simulink model "stm32_system_identification"  (R2025a)
settings: Solver=VariableStepAuto  StartTime=0.0  StopTime=10.0  RelTol=1e-3
values from neighbouring files (symbols this model uses):
  motor_B = 0.000032047    (= 3.2047e-05)    [Lab1_motor_params_student.m]    (also in Params_Chirp.mat = 0.00100006396424; Params_Ramp.mat = 0.301544637419; Params_Sine.mat = 0.229979738857; Params_Stair.mat = 0.140998803706)
  motor_Eff = 0.952868616    [Lab1_motor_params_student.m]    (also in Params_Chirp.mat = 0.999510591885; Params_Ramp.mat = 0.511135750028; Params_Sine.mat = 1; Params_Stair.mat = 0.999629522012)
  motor_J = 0.000009875    (= 9.875e-06)    [Lab1_motor_params_student.m]    (also in Params_Chirp.mat = 0.00100180066555; Params_Ramp.mat = 0.35220653698; Params_Sine.mat = 0.261312099523; Params_Stair.mat = 0.298587602887)
  motor_Ke = 0.047996267    [Lab1_motor_params_student.m]    (also in Params_Chirp.mat = 0.574998179044; Params_Ramp.mat = 0.149481279538; Params_Sine.mat = 0.241485328515; Params_Stair.mat = 0.261815421338)
  motor_L = 0.002853248    [Lab1_motor_params_student.m]
  motor_R = 3.399924458    [Lab1_motor_params_student.m]
undefined symbols (not defined in the file or in its folder): Blocking, LF, Non
libraries: simulink x3, amg_usbconverter_n_connect_lib x3, dspstat3 x1
settings Model: Creator=User  LastModifiedBy=User

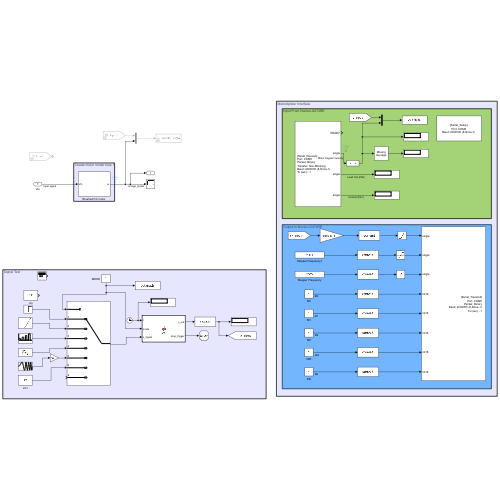
[thumbnail: Simulink's stored preview of the top-level diagram]
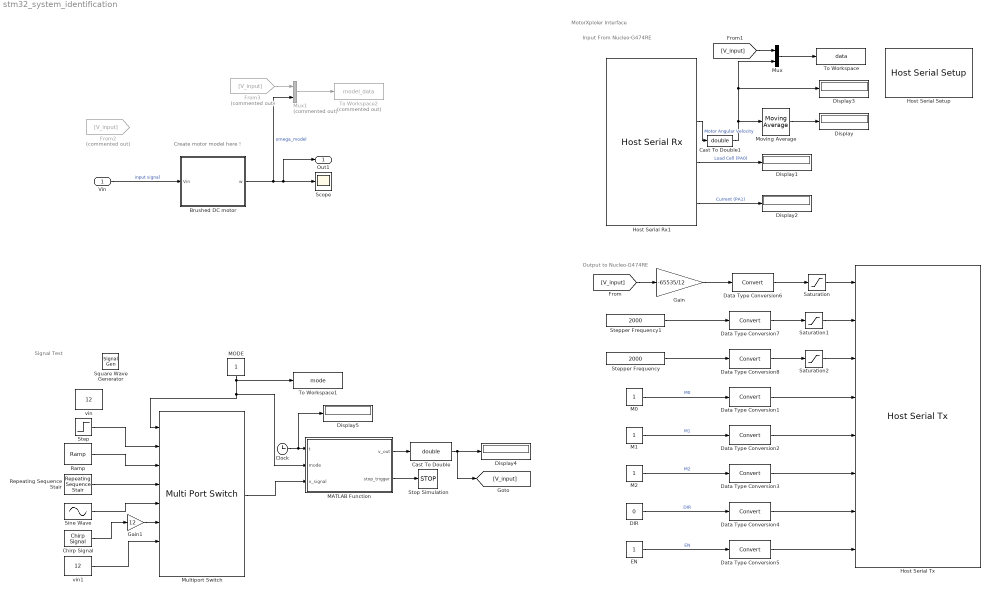
== system stm32_system_identification ==
  note: Signal Test
  note: Input From Nucleo-G474RE
  note: Output to Nucleo-G474RE
  note: MotorXploler Interface
  note: Create motor model here !
  Vin : Inport
  Brushed DC motor : Subsystem
  Cast To Double : DataTypeConversion  OutDataTypeStr=double  SaturateOnIntegerOverflow=off  RndMeth=Floor
  Cast To Double1 : DataTypeConversion  OutDataTypeStr=double  SaturateOnIntegerOverflow=off  RndMeth=Floor
  Chirp Signal : simulink/Sources/Chirp Signal  f1=0  T=20  f2=pi
  Clock : Clock
      settings: Decimation=5
  DIR : Constant  Value=0
  Data Type Conversion{1..8} (8 alike) : DataTypeConversion  SaturateOnIntegerOverflow=off  RndMeth=Floor
  Display{,1..5} (6 alike) : Display
  EN : Constant
  From2 : From  Commented=on  GotoTag=V_input
  From3 : From  Commented=on  GotoTag=V_input
  Gain : Gain  Gain=-65535/12
  Gain1 : Gain  Gain=12
  Host Serial Rx1 : amg_usbconverter_n_connect_lib/Host Serial Rx  conf=rx  port=<auto>  baudrate=2000000  databits=8  parity=None  stopbit=1  flowcontrol=None  transfer=Non-Blocking  timeout=5  packetmode=Binary  enableinitialvalues=off  initialvalues=[]  binheader='25'  binterminator='4E'  porttype_double=0  porttype_single=3  porttype_int8=0  porttype_uint8=0  porttype_int16=0  porttype_uint16=0  porttype_int32=0  porttype_uint32=0  asciiformat='%f,%f,%d,%d'  rx_asciiterminator="LF (0x0A - \"\\n\")"  tx_asciiterminator="CRLF (0x0D 0x0A - \"\\r\\n\")"  sampletime=-1  enablecustomportlabel=off  cinputportlabel=0  coutputportlabel=A  portpinstr=0  blockid=HostSerialRx1  inputporttype=[]  inputportwidth=[]  inputportlabel={}  outputporttype=[3 1 1 1]  outputportwidth=[1 1 1 1]  outputportlabel={'READY','single','single','single'}  compat=0  optionstring=[]  autoport='COM5'
  Host Serial Setup : amg_usbconverter_n_connect_lib/Host Serial Setup  conf=setup  port=<auto>  baudrate=2000000  databits=8  parity=None  stopbit=1  flowcontrol=None  transfer=Blocking  timeout=2  packetmode=Binary  initialvalues=[]  binheader='7E 7E'  binterminator='03 03'  porttype_double=0  porttype_single=1  porttype_int8=0  porttype_uint8=0  porttype_int16=0  porttype_uint16=0  porttype_int32=0  porttype_uint32=2  asciiformat='%d %u %x'  rx_asciiterminator="CRLF (0x0D 0x0A - \"\\r\\n\")"  tx_asciiterminator="CRLF (0x0D 0x0A - \"\\r\\n\")"  sampletime=-1  enablecustomportlabel=off  cinputportlabel=0  coutputportlabel=A  portpinstr=0  blockid=HostSerialSetup  inputporttype=[]  inputportwidth=[]  inputportlabel={}  outputporttype=[]  outputportwidth=[]  outputportlabel={}  compat=0  optionstring=[]  autoport='COM5'
  Host Serial Tx : amg_usbconverter_n_connect_lib/Host Serial Tx  conf=tx  port=<auto>  baudrate=2000000  databits=8  parity=None  stopbit=1  flowcontrol=None  transfer=Blocking  timeout=2  packetmode=Binary  initialvalues=[]  binheader='25'  binterminator='4E'  porttype_double=0  porttype_single=3  porttype_int8=0  porttype_uint8=0  porttype_int16=5  porttype_uint16=0  porttype_int32=0  porttype_uint32=0  asciiformat='%d,%f'  rx_asciiterminator="CRLF (0x0D 0x0A - \"\\r\\n\")"  tx_asciiterminator="CRLF (0x0D 0x0A - \"\\r\\n\")"  sampletime=-1  enablecustomportlabel=off  cinputportlabel=0  coutputportlabel=A  portpinstr=0  blockid=HostSerialTx  inputporttype=[1 1 1 4 4 4 4 4]  inputportwidth=[1 1 1 1 1 1 1 1]  inputportlabel={'single','single','single','int16','int16','int16','int16','int16'}  outputporttype=[]  outputportwidth=[]  outputportlabel={}  compat=0  optionstring=[]  autoport='COM5'
      settings: SourceProductName=aMG USB Converter N
  M0 : Constant
  M1 : Constant
  M2 : Constant
  MATLAB Function : MATLAB Function  TreatAsAtomicUnit=on
  MODE : Constant
  Moving Average : dspstat3/Moving Average  Method=Sliding window  ForgettingFactorPort=off  SpecifyWindowLength=on  WindowLength=4  OverlapLength=3  AllowArbitraryInputLength=off  ForgettingFactor=0.9  SimulateUsing=Interpreted execution
  Multiport Switch : MultiPortSwitch  Inputs=6  DataPortForDefault=Additional data port  SaturateOnIntegerOverflow=off  InputSameDT=off
  Mux : Mux  Inputs=2
  Mux1 : Mux  Commented=on  Inputs=2
  Ramp : simulink/Sources/Ramp  slope=3  start=0  InitialOutput=0
  Repeating Sequence Stair : simulink/Sources/Repeating Sequence Stair  OutValues=[3 0 6 0 9 0 12 0]  tsamp=5  OutMin=[]  OutMax=[]  OutDataTypeStr=double  OutputDataTypeScalingMode=double  OutDataType=fixdt(0,8)  ConRadixGroup=Best Precision: Vector-wise  OutScaling=2^-12
  Saturation : Saturate  UpperLimit=65535  LowerLimit=-65535
  Saturation1 : Saturate  UpperLimit=20000  LowerLimit=0
  Saturation2 : Saturate  UpperLimit=inf  LowerLimit=0
  Scope : Scope
      settings: ActiveDisplayYMinimum=-26.38033  ActiveDisplayYMaximum=237.42293
  Sine Wave : Sin  Amplitude=12  Frequency=pi  SampleTime=0
  Square Wave Generator : SignalGenerator  WaveForm=square  Amplitude=6  Frequency=2000
  Step : Step  After=12  SampleTime=0
  Stepper Frequency : Constant  Value=2000  OutDataTypeStr=single
  Stepper Frequency1 : Constant  Value=2000  OutDataTypeStr=single
  Stop Simulation : Stop
  To Workspace : ToWorkspace  VariableName=data  SaveFormat=Timeseries  SampleTime=-1
  To Workspace1 : ToWorkspace  VariableName=mode  SaveFormat=Timeseries  SampleTime=-1
  To Workspace2 : ToWorkspace  Commented=on  VariableName=model_data  SaveFormat=Timeseries  SampleTime=-1
  vin : Constant  Value=12
  vin1 : Constant  Value=12
  Out1 : Outport
  wires:
  MATLAB Function/2(stop_trigger) -> Stop Simulation/1
  Repeating Sequence Stair/1 -> Multiport Switch/4
  Gain1/1 -> Multiport Switch/6
  Sine Wave/1 -> Multiport Switch/5
  vin1/1 -> Multiport Switch/7
  Step/1 -> Multiport Switch/2
  MATLAB Function/1(v_out) -> Cast To Double/1
  Multiport Switch/1 -> MATLAB Function/3(v_signal)
  Clock/1 -> Display5/1, MATLAB Function/1(t)
  Chirp Signal/1 -> Gain1/1
  Ramp/1 -> Multiport Switch/3
  Cast To Double/1 -> [V_input], Display4/1
  MODE/1 -> Multiport Switch/1, MATLAB Function/2(mode), To Workspace1/1
  Data Type Conversion5/1 -> Host Serial Tx/8
  Host Serial Rx1/4 -> Display2/1  "Current (PA1)"
  Saturation/1 -> Host Serial Tx/1
  M1/1 -> Data Type Conversion2/1  "M1"
  Stepper Frequency1/1 -> Data Type Conversion7/1
  [V_input] -> Gain/1
  Stepper Frequency/1 -> Data Type Conversion8/1
  [V_input] -> Mux/1
  Gain/1 -> Data Type Conversion6/1
  M2/1 -> Data Type Conversion3/1  "M2"
  Data Type Conversion1/1 -> Host Serial Tx/4
  EN/1 -> Data Type Conversion5/1  "EN"
  Host Serial Rx1/3 -> Display1/1  "Load Cell (PA0)"
  DIR/1 -> Data Type Conversion4/1  "DIR"
  Cast To Double1/1 -> Mux/2, Display3/1, Moving Average/1
  Mux/1 -> To Workspace/1
  Data Type Conversion8/1 -> Saturation2/1
  Data Type Conversion4/1 -> Host Serial Tx/7
  Data Type Conversion3/1 -> Host Serial Tx/6
  Host Serial Rx1/2 -> Cast To Double1/1  "Motor Angular Velocity"
  M0/1 -> Data Type Conversion1/1  "M0"
  Moving Average/1 -> Display/1
  Data Type Conversion7/1 -> Saturation1/1
  Saturation2/1 -> Host Serial Tx/3
  Data Type Conversion2/1 -> Host Serial Tx/5
  Saturation1/1 -> Host Serial Tx/2
  Data Type Conversion6/1 -> Saturation/1
  Mux1/1 -> To Workspace2/1
  Brushed DC motor/1(w) -> Mux1/2, Out1/1, Scope/1  "omega_model"
  From3/1 -> Mux1/1
  Vin/1 -> Brushed DC motor/1(Vin)  "input signal"

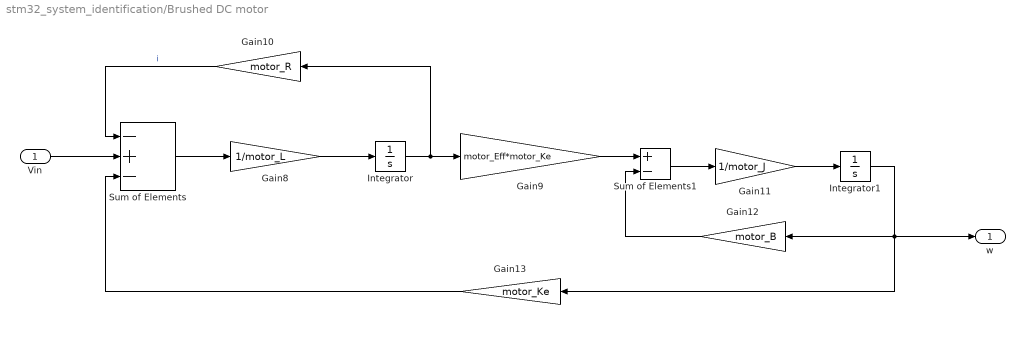
== system stm32_system_identification/Brushed DC motor ==
  Vin : Inport
  Gain10 : Gain  Gain=motor_R
  Gain11 : Gain  Gain=1/motor_J
  Gain12 : Gain  Gain=motor_B
  Gain13 : Gain  Gain=motor_Ke
  Gain8 : Gain  Gain=1/motor_L
  Gain9 : Gain  Gain=motor_Eff*motor_Ke
  Integrator : Integrator
  Integrator1 : Integrator
  Sum of Elements : Sum  Inputs=-+-
  Sum of Elements1 : Sum  Inputs=+-
  w : Outport
  wires:
  Sum of Elements/1 -> Gain8/1
  Gain8/1 -> Integrator/1
  Integrator/1 -> Gain9/1, Gain10/1
  Gain10/1 -> Sum of Elements/1  "i"
  Sum of Elements1/1 -> Gain11/1
  Gain9/1 -> Sum of Elements1/1
  Gain11/1 -> Integrator1/1
  Integrator1/1 -> w/1, Gain13/1, Gain12/1
  Gain12/1 -> Sum of Elements1/2
  Gain13/1 -> Sum of Elements/3
  Vin/1 -> Sum of Elements/2

== matlab function stm32_system_identification/MATLAB Function ==
  data: t input; v_out output; mode input; v_signal input; stop_trigger output
function [v_out, stop_trigger] = fcn(t, mode, v_signal)
    % durations = [Step, Ramp, Stair, Sine, Chirp]
    durations = [3, 4, 40, 10, 20,20]; 
    
    % Stage 1: Running
    if t < durations(mode)
        v_out = v_signal;
        stop_trigger = 0;
        
    % Stage 0: Cutoff and Stop
    else
        v_out = 0;           % Forces the motor to stop immediately
        stop_trigger = 1;    % Triggers the Simulink Stop block
    end
end
